simulink model "vehicle_model"  (R2021b)
settings: Solver=ode23tb  StartTime=0  StopTime=2474  FixedStep=1e-5  RelTol=2e-1
InitFcn:
  | param_v1_script;
  | Ts=0.01;
  | scenario_generator;
  | Regen_on=1;
  | v_nom=10;
values from neighbouring files (symbols this model uses):
  b = 1.504    [dynamics_wheel.m]    (also in param_v1_script.m = Simulink.Parameter)
  BattChargeMax = 4.8    [param_v1_script.m]
  Battery = struct    [param_v1_script.m]
  BattSocInit = 0.75    [param_v1_script.m]
  BattTempInit = 25    [param_v1_script.m]
  BrkPrsMax = 5.0E+6    (= 5000000)    [param_v1_script.m]
  car = vehicle(scenario,'ClassID',1,'Position',[x_ego y_ego 0], 'Yaw' ,0,     'Length',3,'Width',2,'Height',1.6)    [scenario_generator.m]
  disk_abore = 0.05    [param_v1_script.m]
  Eb_init = 54.28*1000*3600    (= 195408000)    [param_v1_script.m]
  efficiency_table = [86.7 86.7 86.7 86.7 86.7 86.7 86.7 86.7 86.7 86.7 86.7 86.7 86.7 86.7     86.7 ... (first row only)    [param_v1_script.m]
  eta_i = 1    [param_v1_script.m]
  Jmotor = Simulink.Parameter    [param_v1_script.m]
  k = Simulink.Parameter    [param_v1_script.m]
  L = 30000    [scenario_generator.m]
  losses_table = [0 0 0 0 0 0 0 0 0 0 0 0 0 0 0 ... (first row only)    [param_v1_script.m]
  m = VEH.Mass    [param_v1_script.m]
  MaxChrgCurrLim = Simulink.Parameter    [param_v1_script.m]
  MaxDchrgCurrLim = Simulink.Parameter    [param_v1_script.m]
  MinCellVoltDchrgCurrentLim_BP = [2.5; 2.75; 3]    [param_v1_script.m]
  MinCellVoltDchrgCurrentLim_Table = [0 0.5 1]    [param_v1_script.m]
  MotSpd = [0 1600 3200 4477.56 4800 6400 8000 9600 11200 12800 14400 16000            ]    [param_v1_script.m]
  MotTrq = [450 450 450 450 419.771162404874 314.828371803655 251.862697442924            209.885581202437 179.901926744946 157.414185901828 139.923720801625            125.931348721462]    [param_v1_script.m]
  mu_kinetic = 0.2    [param_v1_script.m]
  Nd = 7.94    [param_v1_script.m]
  Ndiff = Simulink.Parameter    [param_v1_script.m]
  Np_Module = 31    [param_v1_script.m]
  Ns_Module = 24    [param_v1_script.m]
  num_pads = 2    [param_v1_script.m]
  NumModules = 4    [param_v1_script.m]
  RegenBrkCutOff = [0 1]    [param_v1_script.m]
  RegenBrkSpd_bpt = [5 9]    [param_v1_script.m]
  Rm = 0.177    [param_v1_script.m]
  rw = 0.3345    [param_v1_script.m]
  scenario = drivingScenario('SampleTime',0.1','StopTime',60)    [scenario_generator.m]
  SOCInit = 0.75    [param_v1_script.m]
  SOE_init = SOCInit    (= 0.75)    [param_v1_script.m]
  T_eff_bp = [0 32.142857142857146 64.285714285714292 96.428571428571431              128.57142857142858 160.71428571428572 192.85714285714286 225              257.14285714285717 289.28571428571428 321.42857142857144 353.57142857142856              385.71428571428572 417.85714285714283 450]    [param_v1_script.m]
  threshld = 50    [scenario_generator.m]
  VEH = struct    [dynamics_wheel.m]
  w_eff_bp = [0 1600 3200 4477.56 4800 6400 8000 9600 11200 12800 14400 16000              ]    [param_v1_script.m]
undefined symbols (not defined in the file or in its folder): curvature, direction, DiscIntNeverNeededParam, gradbp, InertFrm, psi_o, thetaRefs, xRef2s, yRef2s
libraries: simulink x11, autolibutils x4, autolibshared x4, autolibsharedcoupling x4, sharedtransform x3, vehdynlibdriver x3, simulink_extras x3, sharedTrackingLibrary x2, vehdynlibtirecommon x2, vehdynlibtire x2, vehdynlibdrivercommon x2, vehdynlibscenariocommon x1
(part 1 of 6)
settings Model: Creator=simran  LastModifiedBy=simran
settings SolverCC: ZeroCrossAlgorithm=Adaptive
settings DebuggingCC: MaskedZcDiagnostic=none  IgnoredZcDiagnostic=none

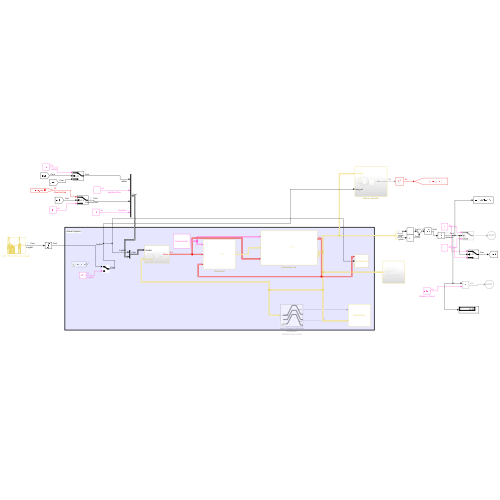
[thumbnail: Simulink's stored preview of the top-level diagram]
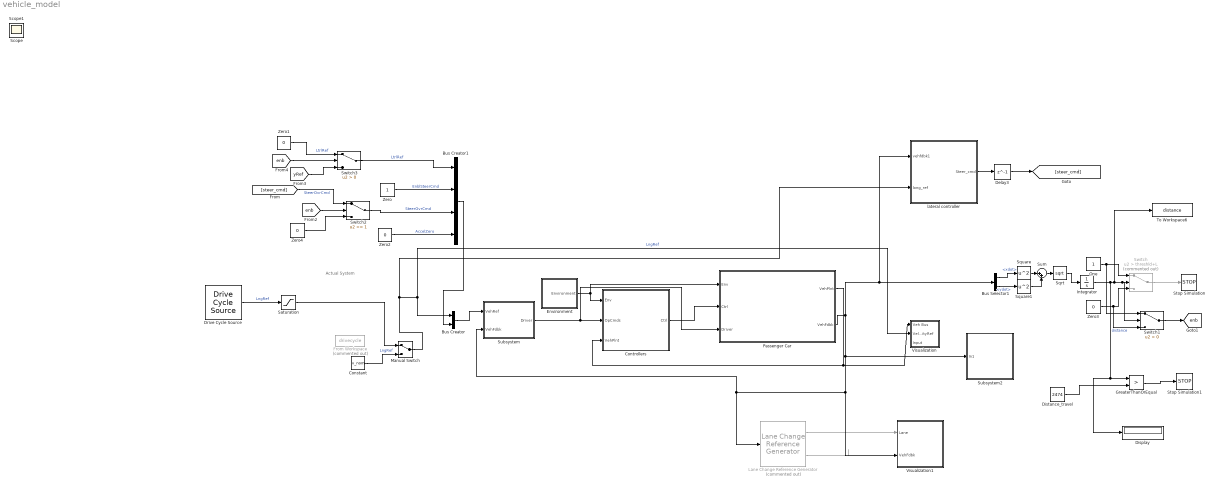
== system vehicle_model ==
  note: Actual System
  Bus Creator : BusCreator  Inputs=2
  Bus Creator1 : BusCreator  Inputs=4
  Bus Selector1 : BusSelector  OutputSignals=Body.BdyFrm.Cg.Vel.xdot,Body.BdyFrm.Cg.Vel.ydot
  Constant : Constant  Value=v_nom
  Controllers : Subsystem
      mask Display: image('SystemControllers.png','center')
  Delay3 : Delay  DelayLength=1
  Display : Display
  Distance_travel : Constant  Value=2474
  Drive Cycle Source : autolibshared/Drive Cycle Source  cycleVar=FTP75  fileVar=L:\Bauto\matlab\test\toolbox\shared\autoblks\scenario\adac.txt  tfinal="2474  seconds"  cycleRepeat=off  outAccPort=off  outGearPort=off  gearList=No gear data  t_wot1=1  xdot_woto=0  xdot_wot1=26.8*1.1  t_wot2=30  xdot_wot2=0  t_wotend=40  srcUnit=m/s  outUnit=m/s  srcAccUnit=m/s/s  outAccUnit=m/s^2  dt=0  aMode=1  faultOption=off  velBnd=2  velBndUnit=mph  inUnit=m/s  timeBnd=1  failOption=off  stopSim=off  maxFaultCnt=10  maxFaultTime=2  maxTotFaultTime=15  traceOption=off  dtTrace=1  traceWindow=10  lastDCname=FTP75  lastOutUnit=mph  lastDT=0  lastTB=1  lastSB=2  forceCalcBound=off
      settings: SourceProductBaseCode=PW,DR,MT,UV,VE
  Environment : Subsystem
      mask Display: disp(getString(message('autoblks:autoblkVehMask:environ')))
  From Workspace : FromWorkspace  Commented=on  VariableName=drivecycle  SampleTime=-1
  GreaterThanOrEqual : RelationalOperator  Operator=>  OutDataTypeStr=boolean  RndMeth=Simplest
  Integrator : Integrator
  Lane Change Reference Generator : vehdynlibscenariocommon/Lane Change Reference Generator  Commented=on  ssMode=Initialize from model  ssVar=dlcSS35mph  t_start=1  XGate=200  xdot_r=35  xdotUnit=mph  xStart=2  vehW=2  latoff=800  lattoff=VEH.InitialLatPosition  centerSwitch=on  xSimStop=off  ssDefault=on  latRefbp=DLCXref  latRef=DLCYref  X_o=175  Y_o=VEH.InitialLatPosition  psi_o=VEH.InitialYawAngle  ssTol=.15  ssMaxTime=30  ssWSName=dlcSS35mph  aMode=2
      link override ISO 3888-2/Lateral Reference: LabelModeActiveChoice=1
      settings: AttributesFormatString=%<ssMode>  SourceProductBaseCode=VE
  Manual Switch : ManualSwitch
  One : Constant  OutDataTypeStr=Inherit: Inherit via back propagation
  Passenger Car : Subsystem
      mask Display: image('PassengerVehicle.png','center')
  Saturation : Saturate  UpperLimit=inf  LowerLimit=5
  Sqrt : Sqrt  SaturateOnIntegerOverflow=on
  Square : Math  Operator=square  SaturateOnIntegerOverflow=on
  Square1 : Math  Operator=square  SaturateOnIntegerOverflow=on
  Stop Simulation : Stop
  Stop Simulation1 : Stop
  Subsystem : Subsystem
  Subsystem2 : Subsystem
  Sum : Sum  Inputs=|++
  Switch : Switch  Commented=on  Criteria=u2 > Threshold  Threshold=threshld+L
  Switch1 : Switch  Criteria=u2 > Threshold
  Switch2 : Switch  Threshold=1
  Switch3 : Switch  Criteria=u2 > Threshold
  To Workspace6 : ToWorkspace  VariableName=distance  SaveFormat=Timeseries  SampleTime=-1
  Visualization : Subsystem
      mask Display: disp(getString(message('autoblks:autoblkVehMask:visual')))
  Visualization1 : Subsystem
      mask Display: disp('Visualization')
  Zero : Constant  OutDataTypeStr=Inherit: Inherit via back propagation
  Zero{1..4} (4 alike) : Constant  Value=0  OutDataTypeStr=Inherit: Inherit via back propagation
  lateral controller : Subsystem
  Scope : Scope
  Scope1 : Scope
  tag scope: enb=global
  wires:
  Lane Change Reference Generator/2 -> ?
  [yRef] -> Switch3/3
  Delay3/1 -> [steer_cmd]
  One/1 -> Switch1/1, Switch/1
  [enb] -> Switch3/2
  Switch1/1 -> [enb]
  lateral controller/1(Steer_cmd) -> Delay3/1
  Integrator/1 -> To Workspace6/1, Switch1/2, Switch/2, Display/1, GreaterThanOrEqual/1  "distance"
  Switch2/1 -> Bus Creator1/3  "SteerOvrCmd"
  Bus Creator1/1 -> Bus Creator/2
  Zero/1 -> Bus Creator1/2  "EnblSteerCmd"
  Bus Creator/1 -> Subsystem/1(VehRef)
  Zero2/1 -> Bus Creator1/4  "AccelZero"
  Switch3/1 -> Bus Creator1/1  "LtrlRef"
  Zero3/1 -> Switch1/3, Switch/3
  Lane Change Reference Generator/1 -> Visualization1/1(Lane)
  Switch/1 -> Stop Simulation/1
  Zero4/1 -> Switch2/3
  Environment/1(Environment) -> Controllers/1(Env), Passenger Car/1(Env)
  Bus Selector1/1 -> Square/1  "<xdot>"
  Passenger Car/2(VehFdbk) -> lateral controller/1(vehfdbk1), Bus Selector1/1, Subsystem/2(VehFdbk), Lane Change Reference Generator/1, Visualization1/2(VehFdbk), Subsystem2/1(In1)
  Manual Switch/1 -> lateral controller/2(long_ref), Visualization/2(VelocityRef), Bus Creator/1  "LngRef"
  Controllers/1(Ctrl) -> Passenger Car/2(Ctrl)
  Zero1/1 -> Switch3/1  "LtrlRef"
  [enb] -> Switch2/2
  Passenger Car/1(VehPlnt) -> Controllers/3(VehPlnt), Visualization/1(Veh Bus)
  Bus Selector1/2 -> Square1/1  "<ydot>"
  Square/1 -> Sum/1
  Square1/1 -> Sum/2
  Sum/1 -> Sqrt/1
  Sqrt/1 -> Integrator/1
  Distance_travel/1 -> GreaterThanOrEqual/2
  GreaterThanOrEqual/1 -> Stop Simulation1/1
  Subsystem/1(Driver) -> Passenger Car/3(Driver), Controllers/2(OpCmds)
  Constant/1 -> Manual Switch/2  "LngRef"
  Drive Cycle Source/1 -> Saturation/1  "LngRef"
  Saturation/1 -> Manual Switch/1
  [steer_cmd] -> Switch2/1  "SteerOvrCmd"

== system vehicle_model/Controllers ==
  Env : Inport
  OpCmds : Inport  Port=2
  VehPlnt : Inport  Port=3
  Powertrain Control Input : Subsystem
  Powertrain Control Module (PCM) : Subsystem
  Powertrain Control Output : Subsystem
  Terminator : Terminator
  Ctrl : Outport  VectorParamsAs1DForOutWhenUnconnected=off
  wires:
  [PtCtrl] -> Ctrl/1
  Env/1 -> Terminator/1
  [OpCmds] -> Powertrain Control Input/1(OpCmds)
  Powertrain Control Output/1(PtCtrl) -> [PtCtrl]
  [VehPlnt] -> Powertrain Control Input/2(VehPlnt)
  VehPlnt/1 -> [VehPlnt]
  OpCmds/1 -> [OpCmds]
  Powertrain Control Input/1(AccelPdl) -> Powertrain Control Module (PCM)/1(AccCmd)
  Powertrain Control Input/2(DecelPdl) -> Powertrain Control Module (PCM)/2(DecCmd)
  Powertrain Control Input/3(VehSpdFdbk) -> Powertrain Control Module (PCM)/3(VehSpdFdbk)
  Powertrain Control Input/4(MotSpd) -> Powertrain Control Module (PCM)/4(MotSpd)
  Powertrain Control Module (PCM)/1(MotTrqCmd) -> Powertrain Control Output/1(MotTrqCmd)
  Powertrain Control Module (PCM)/2(BrakeCmd) -> Powertrain Control Output/2(BrkCmd)
  Powertrain Control Input/5(BMS_Sensors) -> Powertrain Control Module (PCM)/5(BMS_Sensors)
  Powertrain Control Module (PCM)/3(BMS_Info) -> Powertrain Control Output/3(BMS_Info)
  Powertrain Control Module (PCM)/4(BMS_Cmd) -> Powertrain Control Output/4(BMS_Cmd)

== system vehicle_model/Environment ==
  Bus Creator : BusCreator  Inputs=4
  Bus Creator1 : BusCreator  Inputs=4
  Bus Creator2 : BusCreator  Inputs=4
  Bus Creator3 : BusCreator  Inputs=3
  Bus Creator4 : BusCreator  Inputs=3
  Bus Creator5 : BusCreator  Inputs=2
  Constant : Constant  Value=zeros(4,1)
  Constant1 : Constant  Value=ones(4,1)
  Constant2 : Constant  Value=0
  Constant3 : Constant  Value=0
  Constant6 : Constant  Value=300
  Constant7 : Constant  Value=101325
  Demux : Demux
  Demux1 : Demux
  Ground{,1..3} (4 alike) : Ground
  Environment : Outport  VectorParamsAs1DForOutWhenUnconnected=off
  wires:
  Ground2/1 -> Bus Creator5/1  "lam_mu_x"
  Ground3/1 -> Bus Creator5/2  "lam_mu_y"
  Bus Creator2/1 -> Bus Creator4/2  "Ground_mu"
  Bus Creator4/1 -> Bus Creator/3  "Ground"
  Bus Creator3/1 -> Bus Creator/4  "Wind"
  Constant3/1 -> Bus Creator3/1  "wind_x"
  Ground/1 -> Bus Creator3/2  "wind_y"
  Ground1/1 -> Bus Creator3/3  "wind_z"
  Constant6/1 -> Bus Creator/1  "Temp"
  Constant2/1 -> Bus Creator4/1  "Grade"
  Bus Creator/1 -> Environment/1  "Environment"
  Constant7/1 -> Bus Creator/2  "Baro"
  Constant/1 -> Demux/1
  Demux/1 -> Bus Creator1/1  "G_FL_z"
  Demux/2 -> Bus Creator1/2  "G_FR_z"
  Demux/3 -> Bus Creator1/3  "G_RL_z"
  Demux/4 -> Bus Creator1/4  "G_RR_z"
  Bus Creator1/1 -> Bus Creator4/3  "z"
  Constant1/1 -> Demux1/1
  Demux1/1 -> Bus Creator2/1  "mu_FL"
  Demux1/2 -> Bus Creator2/2  "mu_FR"
  Demux1/3 -> Bus Creator2/3  "mu_RL"
  Demux1/4 -> Bus Creator2/4  "mu_RR"

== system vehicle_model/Passenger Car ==
  Env : Inport
  Ctrl : Inport  Port=2
  Driver : Inport  Port=3
  Bus Creator : BusCreator  Inputs=2
  Drivetrain Output : Subsystem
  Drivetrain Plant Input : Subsystem
  Electric Plant Input : Subsystem
  Electric Plant Output : Subsystem
  Subsystem : Subsystem
  Subsystem1 : Subsystem
  Zero-Order Hold : ZeroOrderHold  SampleTime=0.01
  VehPlnt : Outport  VectorParamsAs1DForOutWhenUnconnected=off
  Bus Element Out1 : Outport  Port=2  PortName=VehFdbk  Element=Body
  Bus Element Out2 : Outport  Port=2  PortName=VehFdbk  Element=Wheels
  wires:
  Ctrl/1 -> [Ctrl]
  Env/1 -> [Env], Electric Plant Input/3(Env)  "Env"
  [Ctrl] -> Drivetrain Plant Input/1(Ctrl)
  [VehFdbk] -> Bus Creator/2  "Veh"
  [ElecFdbk] -> Bus Creator/1  "Elec"
  [Ctrl] -> Electric Plant Input/1(Ctrl)  "Ctrl"
  [ElecFdbk] -> Drivetrain Plant Input/2(ElecFdbk)
  [VehFdbk] -> Electric Plant Input/2(Veh)  "Vehfdbk"
  Drivetrain Plant Input/2(BrkCmd) -> Subsystem1/2(BrakeReq)
  Drivetrain Plant Input/1(MotTrq) -> Subsystem1/1(MotTrq)
  Subsystem1/2(MotSpd) -> Drivetrain Output/2(MotSpd)
  Subsystem1/1(vel) -> Drivetrain Output/1(Vel)
  [Env] -> Drivetrain Plant Input/3(Env)
  Drivetrain Plant Input/3(Grade) -> Subsystem1/3(Grade)
  Drivetrain Plant Input/4(WindVel) -> Subsystem1/4(Wind Vel)
  Electric Plant Input/1(MotTrqCmd) -> Subsystem/1(MotTrqCmd)
  Electric Plant Input/2(MotSpd) -> Subsystem/2(MotSpd)
  Electric Plant Input/3(AmbTmp) -> Subsystem/3(AmbTmp)
  Subsystem/2(BattPwr) -> Electric Plant Output/2(BattPwr)
  Subsystem/3(BattCrnt) -> Electric Plant Output/3(BattCrnt)
  Subsystem/4(MotTrq) -> Electric Plant Output/4(MotTrq)
  Subsystem/5(BMS_Sensors) -> Electric Plant Output/5(BMS_Sensors)
  Electric Plant Input/4(BMS_Info) -> Subsystem/4(BMS_Info)
  Subsystem/1(BattSoc) -> Electric Plant Output/1(BattSoc)
  Drivetrain Plant Input/5(mu) -> Subsystem1/5(mu)
  Drivetrain Plant Input/6(Gnd) -> Subsystem1/6(Ground)
  Electric Plant Output/1(ElecFdbk) -> [ElecFdbk]  "Elecfdbk"
  Subsystem1/3(Veh) -> Bus Element Out1/1
  Driver/1 -> Drivetrain Plant Input/4(Driver)  "Drive_input"
  Drivetrain Plant Input/7(Steer) -> Subsystem1/7(Steering)
  Subsystem1/4(Wheels) -> Bus Element Out2/1
  Bus Creator/1 -> Zero-Order Hold/1
  Drivetrain Output/1(VehFdbk) -> [VehFdbk]
  Zero-Order Hold/1 -> VehPlnt/1

== system vehicle_model/Subsystem ==
  VehRef : Inport
  VehFdbk : Inport  Port=2
  Bus Creator1 : BusCreator  Inputs=5
  Bus Selector : BusSelector  OutputSignals=Body.BdyFrm.Cg.Vel.xdot,Body.InertFrm.Cg.Disp.Y,Body.BdyFrm.Cg.Vel.ydot,Body.InertFrm.Cg.Ang.psi,Body.BdyFrm.Cg.AngVel.r,Body.InertFrm.Cg.Disp.X
  Bus Selector1 : BusSelector  OutputSignals=LngRef,signal2.LtrlRef,signal2.EnblSteerCmd,signal2.SteerOvrCmd,signal2.AccelZero
  Cast To Boolean : DataTypeConversion  OutDataTypeStr=boolean
  Constant : Constant  Value=0
  Dead Zone : DeadZone  LowerValue=-.5  UpperValue=.5  ZeroCross=off  SaturateOnIntegerOverflow=on
  From Workspace : FromWorkspace  Commented=on  VariableName=acel  SampleTime=-1
  From Workspace1 : FromWorkspace  Commented=on  VariableName=dcel  SampleTime=-1
  Gain : Gain
  Ground : Ground
  Ground1 : Ground
  Ground2 : Ground
  Longitudinal Driver : autolibshared/Longitudinal Driver  extAccelOvr=off  extDecelOvr=off  extAccelHld=off  extDecelHld=off  extAccelZero=off  extDecelZero=off  cntrlType=PI  shftType=None  velUnits=m/s  gearOut=off  Kp=10  Ki=5  Kff=.1  Kg=0  VehVelVec=[0 100]  KffVec=[.1 .1]  KpVec=[10 10]  KiVec=[5 5]  KgVec=[0 0]  m=1500  Kpt=3000  tau=.1  L=2  aR=200  bR=2.5  cR=.5  g=9.81  vnom=10  Kaw=1  tauerr=.01  tauPt=2  GearInit=0  tShift=.1  pdlVec=[0.1 0.4 0.5 0.9]  upShftTbl=[-1 12.9375 26.4375 39.9375 51.18749999999999 62.4375 72.84375 83.25;-1 16.3125 29.8125 43.3125 54.5624 65.8125 76.78125 87.75;-1 19.6875 33.1875 46.68749999999999 57.9375 69.1875 80.71875 92.25;-1 33 52.5 77.25 100.5 138.75 161.875 185]  dwnShftTbl=[1 9.5625 23.0625 36.5625 47.8125 59.0625 68.90625 78.75;1 12.9375 26.4375 39.9375 51.18749999999999 62.4375 72.84375 83.25;1 16.3125 29.8125 43.3125 54.562499 65.8125 76.78125 87.75;1 19.6875 33.1875 46.68749999999999 57.9375 69.1875 80.71875 92.25]  tClutch=.5  tRev=.5  tPark=120  aMode=2  UpGearVec="[0  1  2  3  4  5  6  7]"  DownGearVec="[1  2  3  4  5  6  7  8]"
      settings: SourceProductBaseCode=PW,DR,MT,UV,VE
  Mux : Mux  Inputs=3
  Subsystem : Subsystem  Commented=on
  Terminator1 : Terminator
  Terminator2 : Terminator
  Zero : Constant  Value=0  OutDataTypeStr=Inherit: Inherit via back propagation
  Zero-Order Hold : ZeroOrderHold  SampleTime=Ts
  Zero1 : Constant  Value=0  OutDataTypeStr=Inherit: Inherit via back propagation
  Driver : Outport  VectorParamsAs1DForOutWhenUnconnected=off
  wires:
  Dead Zone/1 -> Longitudinal Driver/2, Subsystem/6(VelFdbk)
  Bus Selector1/1 -> Subsystem/1(VelRef), Longitudinal Driver/1  "<LngRef>"
  Bus Selector1/4 -> Gain/1, Subsystem/3(SteerOvrCmd)  "<SteerOvrCmd>"
  Bus Selector1/3 -> Subsystem/4(EnblSteerOvr)  "<EnblSteerCmd>"
  VehRef/1 -> Bus Selector1/1  "xdotref"
  VehFdbk/1 -> Bus Selector/1
  Zero1/1 -> Mux/3
  Longitudinal Driver/2 -> Bus Creator1/2  "AccelCmd"
  Bus Selector/3 -> Subsystem/8(LatVelFdbk)  "<ydot>"
  Bus Selector/4 -> Subsystem/9(YawFdbk)  "<psi>"
  Zero/1 -> Subsystem/7(LatFdbk)
  Bus Creator1/1 -> Zero-Order Hold/1
  Bus Selector/5 -> Subsystem/10(YawVelFdbk)  "<r>"
  Ground/1 -> Subsystem/5(Grade)
  Longitudinal Driver/3 -> Bus Creator1/3  "DecelCmd"
  Bus Selector/1 -> Dead Zone/1  "<xdot>"
  Bus Selector1/2 -> Subsystem/2(LatRef), Mux/2  "<LtrlRef>"
  Ground2/1 -> Bus Creator1/4  "GearCmd"
  Bus Selector/6 -> Mux/1  "<X>"
  Mux/1 -> Bus Creator1/5  "Ref"
  Subsystem/1(Info) -> Terminator1/1
  Constant/1 -> Cast To Boolean/1
  Ground1/1 -> Longitudinal Driver/3
  Longitudinal Driver/1 -> Terminator2/1
  Gain/1 -> Bus Creator1/1  "SteerCmd"
  Zero-Order Hold/1 -> Driver/1

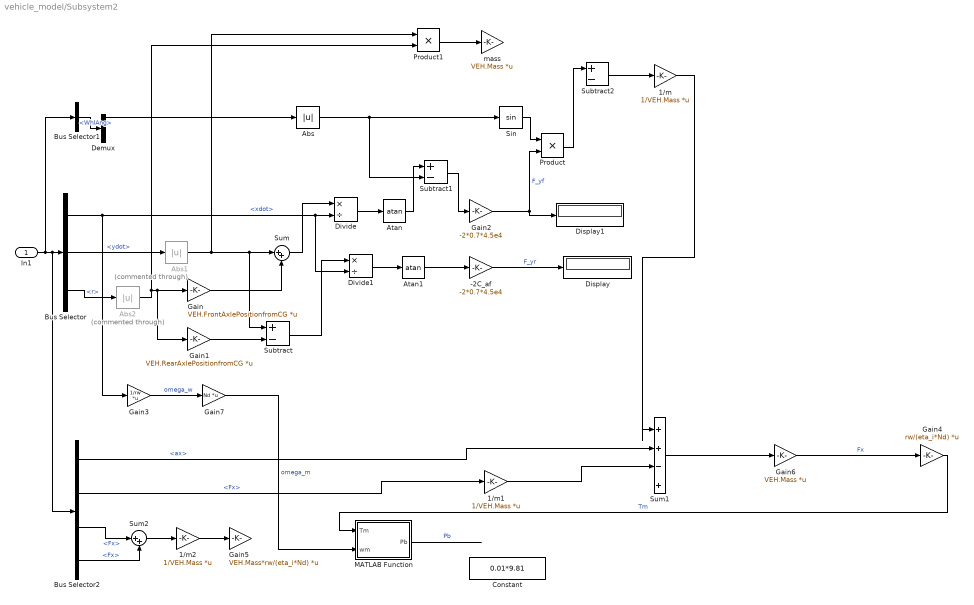
== system vehicle_model/Subsystem2 ==
  In1 : Inport
  -2C_af : Gain  Gain=-2*0.7*4.5e4
  1/m : Gain  Gain=1/VEH.Mass  Multiplication=Matrix(K*u)
  1/m1 : Gain  Gain=1/VEH.Mass  Multiplication=Matrix(K*u)
  1/m2 : Gain  Gain=1/VEH.Mass  Multiplication=Matrix(K*u)
  Abs : Abs
  Abs1 : Abs  Commented=through
  Abs2 : Abs  Commented=through
  Atan : Trigonometry  Operator=atan
  Atan1 : Trigonometry  Operator=atan
  Bus Selector : BusSelector  OutputSignals=Body.BdyFrm.Cg.Vel.xdot,Body.BdyFrm.Cg.Vel.ydot,Body.BdyFrm.Cg.AngVel.r
  Bus Selector1 : BusSelector  OutputSignals=Wheels.signal1.Steering.WhlAng
  Bus Selector2 : BusSelector  OutputSignals=Body.BdyFrm.Cg.Acc.ax,Body.BdyFrm.Forces.Drag.Fx,Body.BdyFrm.Forces.RearAxl.Lft.Fx,Body.BdyFrm.Forces.RearAxl.Rght.Fx
  Constant : Constant  Value=0.01*9.81
  Demux : Demux
  Display : Display
  Display1 : Display
  Divide : Product  Inputs=*/
  Divide1 : Product  Inputs=*/
  Gain : Gain  Gain=VEH.FrontAxlePositionfromCG  Multiplication=Matrix(K*u)
  Gain1 : Gain  Gain=VEH.RearAxlePositionfromCG  Multiplication=Matrix(K*u)
  Gain2 : Gain  Gain=-2*0.7*4.5e4
  Gain3 : Gain  Gain=1/rw  Multiplication=Matrix(K*u)
  Gain4 : Gain  Gain=rw/(eta_i*Nd)  Multiplication=Matrix(K*u)
  Gain5 : Gain  Gain=VEH.Mass*rw/(eta_i*Nd)  Multiplication=Matrix(K*u)
  Gain6 : Gain  Gain=VEH.Mass  Multiplication=Matrix(K*u)
  Gain7 : Gain  Gain=Nd  Multiplication=Matrix(K*u)
  MATLAB Function : MATLAB Function  TreatAsAtomicUnit=on
  Product : Product
  Product1 : Product
  Sin : Trigonometry
  Subtract : Sum  Inputs=+-
  Subtract1 : Sum  Inputs=+-
  Subtract2 : Sum  Inputs=+-
  Sum : Sum  Inputs=|++
  Sum1 : Sum  Inputs=|++-+
  Sum2 : Sum  Inputs=|++
  mass : Gain  Gain=VEH.Mass  Multiplication=Matrix(K*u)
  wires:
  In1/1 -> Bus Selector1/1, Bus Selector2/1, Bus Selector/1
  Bus Selector/2 -> Abs1/1  "<ydot>"
  Bus Selector/3 -> Abs2/1  "<r>"
  Gain/1 -> Sum/2
  Gain1/1 -> Subtract/2
  Sum/1 -> Divide/1
  Bus Selector/1 -> Gain3/1, Divide/2, Divide1/2  "<xdot>"
  Subtract/1 -> Divide1/1
  Divide/1 -> Atan/1
  Divide1/1 -> Atan1/1
  Atan1/1 -> -2C_af/1
  Atan/1 -> Subtract1/1
  Gain2/1 -> Product/2, Display1/1  "F_yf"
  -2C_af/1 -> Display/1  "F_yr"
  Bus Selector1/1 -> Demux/1  "<WhlAng>"
  Demux/1 -> Abs/1
  Subtract1/1 -> Gain2/1
  Gain7/1 -> MATLAB Function/2(wm)  "omega_m"
  Sin/1 -> Product/1
  Product1/1 -> mass/1
  Product/1 -> Subtract2/1
  Subtract2/1 -> 1/m/1
  1/m1/1 -> Sum1/3
  Bus Selector2/1 -> Sum1/2  "<ax>"
  1/m/1 -> Sum1/1
  Sum1/1 -> Gain6/1
  Bus Selector2/3 -> Sum2/1  "<Fx>"
  Bus Selector2/4 -> Sum2/2  "<Fx>"
  Sum2/1 -> 1/m2/1
  1/m2/1 -> Gain5/1
  Gain4/1 -> MATLAB Function/1(Tm)  "Tm"
  MATLAB Function/1(Pb) -> ?  "Pb"
  Abs/1 -> Sin/1, Subtract1/2
  Abs1/1 -> Product1/1, Subtract/1, Sum/1
  Abs2/1 -> Gain1/1, Gain/1, Product1/2
  Gain3/1 -> Gain7/1  "omega_w"
  Bus Selector2/2 -> 1/m1/1  "<Fx>"
  Gain6/1 -> Gain4/1  "Fx"

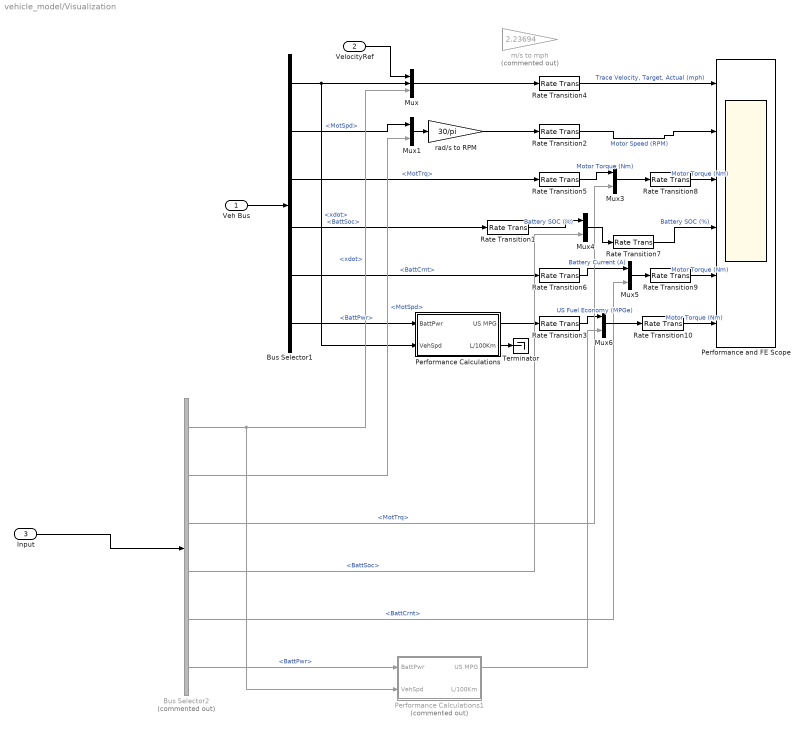
== system vehicle_model/Visualization ==
  Veh Bus : Inport
  VelocityRef : Inport  Port=2
  Input : Inport  Port=3
  Bus Selector1 : BusSelector  OutputSignals=Veh.xdot,Veh.MotSpd,Elec.MotTrq,Elec.BattSoc,Elec.BattCrnt,Elec.BattPwr
  Bus Selector2 : BusSelector  Commented=on  OutputSignals=Veh.xdot,Veh.MotSpd,Elec.MotTrq,Elec.BattSoc,Elec.BattCrnt,Elec.BattPwr
  Mux : Mux  Inputs=3
  Mux{1,3..6} (5 alike) : Mux  Inputs=2
  Performance Calculations : Subsystem
  Performance Calculations1 : Subsystem  Commented=on
  Performance and FE Scope : Scope  NumInputPorts=6
  Rate Transition{1..10} (10 alike) : RateTransition  Deterministic=off
  Terminator : Terminator
  m/s to mph : Gain  Commented=on  Gain=2.23694
  rad/s to RPM : Gain  Gain=30/pi
  wires:
  Veh Bus/1 -> Bus Selector1/1
  Bus Selector1/1 -> Performance Calculations/2(VehSpd), Mux/2  "<xdot>"
  Performance Calculations/1(US MPG) -> Rate Transition3/1
  Performance Calculations/2(L/100Km) -> Terminator/1
  Mux/1 -> Rate Transition4/1
  Bus Selector1/4 -> Rate Transition1/1  "<BattSoc>"
  VelocityRef/1 -> Mux/1
  Rate Transition1/1 -> Mux4/1  "Battery SOC (%)"
  Rate Transition2/1 -> Performance and FE Scope/2  "Motor Speed (RPM)"
  Rate Transition4/1 -> Performance and FE Scope/1  "Trace Velocity, Target, Actual (mph)"
  Bus Selector1/2 -> Mux1/1  "<MotSpd>"
  Bus Selector1/6 -> Performance Calculations/1(BattPwr)  "<BattPwr>"
  rad/s to RPM/1 -> Rate Transition2/1
  Bus Selector1/3 -> Rate Transition5/1  "<MotTrq>"
  Rate Transition5/1 -> Mux3/1  "Motor Torque (Nm)"
  Rate Transition6/1 -> Mux5/1  "Battery Current (A)"
  Bus Selector1/5 -> Rate Transition6/1  "<BattCrnt>"
  Rate Transition3/1 -> Mux6/1  "US Fuel Economy (MPGe)"
  Input/1 -> Bus Selector2/1
  Bus Selector2/1 -> Performance Calculations1/2(VehSpd), Mux/3  "<xdot>"
  Bus Selector2/2 -> Mux1/2  "<MotSpd>"
  Mux3/1 -> Rate Transition8/1
  Bus Selector2/3 -> Mux3/2  "<MotTrq>"
  Mux4/1 -> Rate Transition7/1
  Bus Selector2/4 -> Mux4/2  "<BattSoc>"
  Mux5/1 -> Rate Transition9/1
  Bus Selector2/5 -> Mux5/2  "<BattCrnt>"
  Mux6/1 -> Rate Transition10/1
  Mux1/1 -> rad/s to RPM/1
  Bus Selector2/6 -> Performance Calculations1/1(BattPwr)  "<BattPwr>"
  Performance Calculations1/1(US MPG) -> Mux6/2
  Rate Transition7/1 -> Performance and FE Scope/4  "Battery SOC (%)"
  Rate Transition8/1 -> Performance and FE Scope/3  "Motor Torque (Nm)"
  Rate Transition9/1 -> Performance and FE Scope/5  "Motor Torque (Nm)"
  Rate Transition10/1 -> Performance and FE Scope/6  "Motor Torque (Nm)"

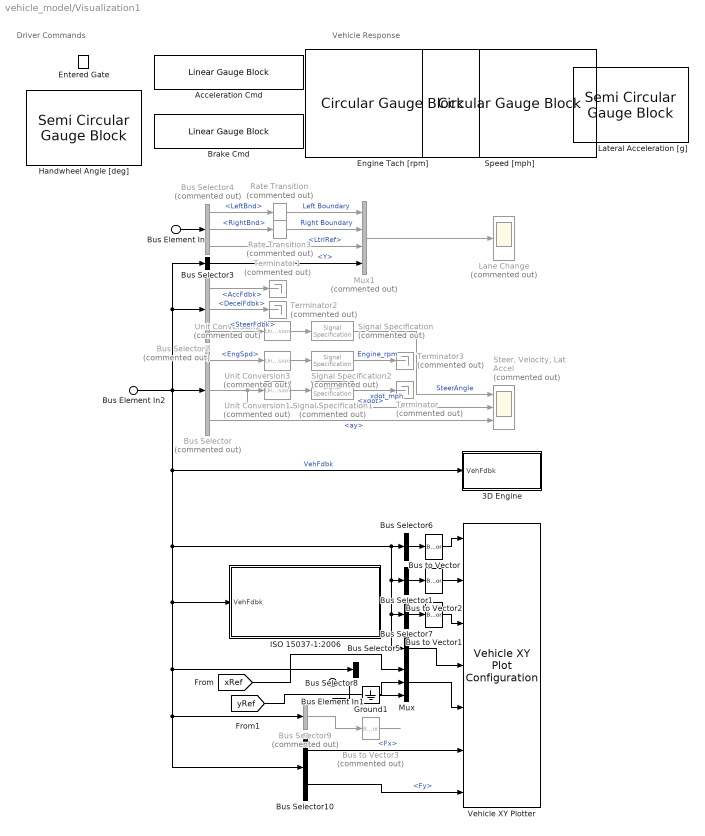
== system vehicle_model/Visualization1 ==
  note: Vehicle Response
  note: Driver Commands
  Bus Element In : Inport  PortName=Lane
  Bus Element In1 : Inport  PortName=Lane  Element=LtrlRef
  Bus Element In2 : Inport  Port=2  PortName=VehFdbk
  3D Engine : Subsystem  Variant=on  mask(3D Engine){engine3D=Disabled, use3DOp=off, SceneDesc=Double lane change, dt3D=.03, defaultPos=Recommended for scene, X_o=0, Y_o=3.125, Z_o=0, phi_o=0, theta_o=0, psi_o=0}
      mask prompts: engine3D "3D Engine"; use3DOp "Use default operating point"; SceneDesc "Scene:"; dt3D "Engine frame rate, dt3D [s]:"; X_o "Initial longitudinal position, X_o [m]:"; Y_o "Initial lateral position, Y_o [m]:"; Z_o "Initial vertical position, Z_o [m]:"; phi_o "Initial roll angle, phi_o [rad]:"; theta_o "Initial pitch angle, theta_o [rad]:"; psi_o "Initial yaw angle, psi_o [rad]:"
      mask help: This subsystem contains the interface blocks which permit the display of the vehicle in the 3D virtual environment. Enable it to view the simulation progress, disable it to inhibit the display.
      mask init:
      | switch get_param(gcb,'engine3D')
      |     case 'Disabled'
      |         try
      |             set_param([bdroot '/Environment/Ground Feedback'],'OverrideUsingVariant','0');
      |         catch
      |             disp('Warning: No ground feedback sensor not set')
      |         end
      |         try
      |             if strcmp(get_param(gcb,'use3DOp'),'on') && strcmp(get_param('DLCReferenceApplication/Lane Change Reference Generator','ssMode'),'Resume from a workspace variable')
      |                 set_param('DLCReferenceApplication/Lane Change Reference Generator','ssVar','dlcSS35mph');
      |             end
      |         catch
      |              disp('Warning: Lane Change Reference Generator not found. Steady state operating point not set')
      |         end
      |     case 'Enabled'
      |         try
      |             set_param([bdroot '/Environment/Ground Feedback'],'OverrideUsingVariant','1');            
      |         catch
      |             disp('Warning: No ground feedback sensor not set')
      |         end
      |         try
      |             if strcmp(get_param(gcb,'use3DOp'),'on') && strcmp(get_param('DLCReferenceApplication/Lane Change Reference Generator','ssMode'),'Resume from a workspace variable')
      |                 set_param('DLCReferenceApplication/Lane Change Reference Generator','ssVar','dlcSS35mph3D');
      |             end
      |         catch
      |              disp('Warning: Lane Change Reference Generator not found. Steady state operating point not set')
      |         end
      |     otherwise
      | end
      settings: AttributesFormatString=|
      | %<SceneDesc>
      | %<engine3D>
      mask Help: eval('vdynblkshelp(''vdynblks3dengine'')');
      mask TypeOptions engine3D: Enabled | Disabled
      mask TypeOptions SceneDesc: 3D Engine/Simulation 3D Scene Configuration/SceneDesc
      mask Callback SceneDesc:
      | defaultStatus = get_param(gcb,'defaultPos');
      | if strcmp(defaultStatus,'Recommended for scene')
      | sceneType = get_param(gcb,'SceneDesc');
      | switch sceneType
      |     case 'Straight road'
      |         set_param(gcb,'X_o', '-118')
      |         set_param(gcb,'Y_o', '3.125')
      |         set_param(gcb,'Z_o', '0')
      |         set_param(gcb,'phi_o', '0')
      |         set_param(gcb,'theta_o', '0')
      |         set_param(gcb,'psi_o', '0')
      |     case 'Curved road'
      |         set_param(gcb,'X_o', '0.2')
      |         set_param(gcb,'Y_o', '-1605.0')
      |         set_param(gcb,'Z_o', '0')
      |         set_param(gcb,'phi_o', '0')
      |         set_param(gcb,'theta_o', '0')
      |         set_param(gcb,'psi_o', '-156*pi/180')
      |     case 'Parking lot'
      |         set_param(gcb,'X_o', '-104.0')
      |         set_param(gcb,'Y_o', '-9.7')
      |         set_param(gcb,'Z_o', '0')
      |         set_param(gcb,'phi_o', '0')
      |         set_param(gcb,'theta_o', '0')
      |         set_param(gcb,'psi_o', '0')
      |     case 'Double lane change'
      |         set_param(gcb,'X_o', '0')
      |         set_param(gcb,'Y_o', '3.125')
      |         set_param(gcb,'Z_o', '0')
      |         set_param(gcb,'phi_o', '0')
      |         set_param(gcb,'theta_o', '0')
      |         set_param(gcb,'psi_o', '0')
      |     case 'Open surface'
      |         set_param(gcb,'X_o', '0')
      |         set_param(gcb,'Y_o', '0')
      |         set_param(gcb,'Z_o', '0')
      |         set_param(gcb,'phi_o', '0')
      |         set_param(gcb,'theta_o', '0')
      |         set_param(gcb,'psi_o', '0')
      |     case 'US highway'
      |         set_param(gcb,'X_o', '3592.00')
      |         set_param(gcb,'Y_o', '2617.00')
      |         set_param(gcb,'Z_o', '-1.0')
      |         set_param(gcb,'phi_o', '0')
      |         set_param(gcb,'theta_o', '0')
      |         set_param(gcb,'psi_o', '0')
      |     case 'US city block'
      |         set_param(gcb,'X_o', '-125.19')
      |         set_param(gcb,'Y_o', '1.65')
      |         set_param(gcb,'Z_o', '-0.04')
      |         set_param(gcb,'phi_o', '0')
      |         set_param(gcb,'theta_o', '0')
      |         set_param(gcb,'psi_o', '0')
      |     case 'Large parking lot'
      |         set_param(gcb,'X_o', '45.0')
      |         set_param(gcb,'Y_o', '54.7')
      |         set_param(gcb,'Z_o', '0.0')
      |         set_param(gcb,'phi_o', '0')
      |         set_param(gcb,'theta_o', '0')
      |         set_param(gcb,'psi_o', '-pi/2')
      |     case 'Virtual Mcity'
      |         set_param(gcb,'X_o', '-26.0')
      |         set_param(gcb,'Y_o', '76.0')
      |         set_param(gcb,'Z_o', '0.0')
      |         set_param(gcb,'phi_o', '0')
      |         set_param(gcb,'theta_o', '0')
      |         set_param(gcb,'psi_o', '-40*pi/180')
      |     otherwise
      |         set_param(gcb,'X_o', '0')
      |         set_param(gcb,'Y_o', '0')
      |         set_param(gcb,'Z_o', '0')
      |         set_param(gcb,'phi_o', '0')
      |         set_param(gcb,'theta_o', '0')
      |         set_param(gcb,'psi_o', '0')
      | end
      | end
      mask TypeOptions defaultPos: Recommended for scene | User-specified
      mask DialogControl engineConfig Prompt: 3D Engine Settings
      mask DialogControl posSetup Prompt: Initial vehicle position
      mask DialogControl posSetupDesc Prompt: To use these initial vehicle positions, first Apply the initial values and then click Update the model workspaces with the initial values.
      mask DialogControl setModelPos Prompt: Update model workspaces with initial values
      mask DialogControl setModelPos Callback:
      | if strcmp(get_param(bdroot(gcb),'SimulationStatus'),'stopped')
      |     sceneType = get_param(gcb,'SceneDesc');
      |     rootModel = bdroot(gcb);
      |     ws = get_param(rootModel, 'modelworkspace');
      |     VEH = getVariable(ws,'VEH');
      |     ParamList={'X_o',[1,1],{};'Y_o',[1,1],{};'Z_o',[1,1],{};'phi_o',[1,1],{'gte',-pi/2;'lte',pi/2};'theta_o',[1,1],{'gte',-pi/2;'lte',pi/2};'psi_o',[1,1],{'gte',-2*pi;'lte',2*pi}};
      |     paramStruct = autoblkscheckparams(gcb, '3D Engine',ParamList);
      |     VEH.InitialLongPosition = paramStruct.X_o;
      |     VEH.InitialLatPosition = paramStruct.Y_o;
      |     VEH.InitialVertPosition = paramStruct.Z_o;
      |     VEH.InitialRollAngle = paramStruct.phi_o;
      |     VEH.InitialPitchAngle = paramStruct.theta_o;
      |     VEH.InitialYawAngle = paramStruct.psi_o;
      |     assignin(ws,'VEH',VEH);
      |     modelList = {'PassVeh14DOF','PassVeh7DOF'};
      |     for idx =1:length(modelList)
      | %         try
      |             load_system(modelList{idx});
      |             ws = get_param(modelList{idx}, 'modelworkspace');
      |             assignin(ws,'VEH',VEH);
      |             save_system(modelList{idx});
      |             close_system(modelList{idx});
      | %         catch
      | %             disp(['Cannot find ' modelList{idx}])
      | %         end
      |     end
      | end
      mask Display: disp('3D Engine')
  Acceleration Cmd : LinearGaugeBlock  LabelPosition=Hide  ScaleMax=1  TickInterval=0.20000000000000001
  Brake Cmd : LinearGaugeBlock  LabelPosition=Hide  ScaleMax=1  TickInterval=0.20000000000000001
  Bus Selector : BusSelector  Commented=on  OutputSignals=Driveline.EngSpd,Body.BdyFrm.Cg.Vel.xdot,Body.BdyFrm.Cg.Acc.ay
  Bus Selector1 : BusSelector  OutputSignals=Body.InertFrm.Cg.Ang.phi,Body.InertFrm.Cg.Ang.theta,Body.InertFrm.Cg.Ang.psi  OutputAsBus=on
  Bus Selector10 : BusSelector  OutputSignals=Wheels.signal1.TireFrame.Fx,Wheels.signal1.TireFrame.Fy
  Bus Selector2 : BusSelector  Commented=on  OutputSignals=Driver.AccFdbk,Driver.DecelFdbk,Driver.SteerFdbk
  Bus Selector3 : BusSelector  OutputSignals=Body.InertFrm.Cg.Disp.Y
  Bus Selector4 : BusSelector  Commented=on  OutputSignals=LeftBnd,RightBnd,LtrlRef
  Bus Selector5 : BusSelector  OutputSignals=Wheels.signal1.Steering.WhlAng  OutputAsBus=on
  Bus Selector6 : BusSelector  OutputSignals=Body.InertFrm.Geom.Disp.X,Body.InertFrm.Geom.Disp.Y,Body.InertFrm.Geom.Disp.Z  OutputAsBus=on
  Bus Selector7 : BusSelector  OutputSignals=Body.InertFrm.Geom.Vel.Xdot,Body.InertFrm.Geom.Vel.Ydot,Body.InertFrm.Geom.Vel.Zdot  OutputAsBus=on
  Bus Selector8 : BusSelector  OutputSignals=Body.InertFrm.Cg.Disp.X
  Bus Selector9 : BusSelector  Commented=on  OutputSignals=Driveline.EngSpd,Driveline.Gear  OutputAsBus=on
  Bus to Vector : BusToVector
  Bus to Vector1 : BusToVector
  Bus to Vector2 : BusToVector
  Bus to Vector3 : BusToVector  Commented=on
  Engine Tach [rpm] : CircularGaugeBlock  LabelPosition=Hide  ScaleMax=8000  TickInterval=1000
  Entered Gate : LampBlock  LabelPosition=Hide
  Ground1 : Ground
  Handwheel Angle [deg] : SemiCircularGaugeBlock  LabelPosition=Hide  ScaleMin=-300  ScaleMax=300  TickInterval=60
  ISO 15037-1:2006 : Subsystem  StopFcn=|  Variant=on  VariantControlMode=label  LabelModeActiveChoice=0  mask(ISO 15037-1:2006){Measurement=Disabled}
      | switch get_param(gcb,'Measurement')
      |     case 'Enabled'
      |        p=slproject.getCurrentProject;
      |        projectRoot=p.RootFolder;
      |        SySFolder=fullfile(projectRoot, 'System');
      |        Simulink.sdi.loadView([SySFolder filesep 'ISO15037_1_2006E.mldatx']);
      |        Simulink.sdi.view;
      | end
      mask prompts: Measurement "ISO Measurements"
      mask help: Enables display of ISO 15037-1:2006 standard measurement signals in the Simulation Data Inspector.
      mask init:
      | switch get_param(gcb,'Measurement')
      |     case 'Disabled'
      |         set_param(gcb,'OverrideUsingVariant','0')
      |     case 'Enabled'
      |        set_param(gcb,'OverrideUsingVariant','1')
      |     otherwise
      |        set_param(gcb,'OverrideUsingVariant','0')
      | end
      settings: AttributesFormatString=%<Measurement>
      mask Help: eval('vdynblkshelp(''iso15037'')');
      mask TypeOptions Measurement: Enabled | Disabled
      mask Callback Measurement:
      | switch get_param(gcb,'Measurement')
      |     case 'Disabled'
      |         set_param(gcb,'OverrideUsingVariant','0')
      |     case 'Enabled'
      |        set_param(gcb,'OverrideUsingVariant','1')
      |     otherwise
      |        set_param(gcb,'OverrideUsingVariant','0')
      | end
      mask Display: disp('ISO 15037-1:2006')
  Lane Change : Scope  Commented=on
  Lateral Acceleration [g] : SemiCircularGaugeBlock  LabelPosition=Hide  ScaleMin=-1  ScaleMax=1  TickInterval=0.5
  Mux : Mux  Inputs=3
  Mux1 : Mux  Commented=on
  Rate Transition : RateTransition  Commented=on  OutPortSampleTime=.1
  Rate Transition3 : RateTransition  Commented=on  OutPortSampleTime=.1
  Signal Specification : SignalSpecification  Commented=on  Unit=deg
  Signal Specification1 : SignalSpecification  Commented=on  Unit=mph
  Signal Specification2 : SignalSpecification  Commented=on  Unit=rpm
  Speed [mph] : CircularGaugeBlock  LabelPosition=Hide  TickInterval=10
  "Steer, Velocity, Lat Accel" : Scope  Commented=on  NumInputPorts=3
  Terminator{,1..3} (4 alike) : Terminator  Commented=on
  Unit Conversion1 : UnitConversion  Commented=on
  Unit Conversion2 : UnitConversion  Commented=on
  Unit Conversion3 : UnitConversion  Commented=on
  Vehicle XY Plotter : vehdynlibviscommon/Vehicle XY Plot Configuration  extRef=on  extStats=off  extTireF=on  a=VEH.FrontAxlePositionfromCG  b=VEH.RearAxlePositionfromCG  w=VEH.TrackWidth  figBorder=10  bufferSize=1024  velNorm=5  tireFNorm=1000  pltDT=.1
      settings: SourceProductBaseCode=VE
  wires:
  Signal Specification/1 -> "Steer, Velocity, Lat Accel"/1  "SteerAngle"
  Bus Selector/3 -> "Steer, Velocity, Lat Accel"/3  "<ay>"
  Bus Selector/2 -> "Steer, Velocity, Lat Accel"/2, Unit Conversion1/1  "<xdot>"
  Unit Conversion2/1 -> Signal Specification/1
  Unit Conversion1/1 -> Signal Specification1/1
  Signal Specification1/1 -> Terminator/1  "xdot_mph"
  Bus Selector4/2 -> Rate Transition3/1  "<RightBnd>"
  Mux1/1 -> Lane Change/1
  Bus Selector3/1 -> Mux1/4  "<Y>"
  Bus Selector4/1 -> Rate Transition/1  "<LeftBnd>"
  Bus Selector4/3 -> Mux1/3  "<LtrlRef>"
  Bus Selector2/3 -> Unit Conversion2/1  "<SteerFdbk>"
  Bus Selector2/1 -> Terminator1/1  "<AccFdbk>"
  Bus Selector2/2 -> Terminator2/1  "<DecelFdbk>"
  Signal Specification2/1 -> Terminator3/1  "Engine_rpm"
  Unit Conversion3/1 -> Signal Specification2/1
  Bus Selector/1 -> Unit Conversion3/1  "<EngSpd>"
  Bus Selector7/1 -> Bus to Vector1/1
  Bus to Vector/1 -> Vehicle XY Plotter/1
  Bus Selector6/1 -> Bus to Vector/1
  Bus to Vector1/1 -> Vehicle XY Plotter/3
  Bus Selector1/1 -> Bus to Vector2/1
  Bus Element In2/1 -> ISO 15037-1:2006/1(VehFdbk), Bus Selector10/1, Bus Selector9/1, Bus Selector8/1, Bus Selector5/1, Bus Selector7/1, Bus Selector1/1, Bus Selector6/1, 3D Engine/1(VehFdbk), Bus Selector3/1, Bus Selector2/1, Bus Selector/1  "VehFdbk"
  Mux/1 -> Vehicle XY Plotter/5
  Ground1/1 -> Mux/3
  Bus Element In/1 -> Bus Selector4/1
  Bus Element In1/1 -> ?
  Bus to Vector3/1 -> ?
  Bus Selector9/1 -> Bus to Vector3/1
  Bus to Vector2/1 -> Vehicle XY Plotter/2
  Bus Selector5/1 -> Vehicle XY Plotter/4
  Bus Selector10/2 -> Vehicle XY Plotter/7  "<Fy>"
  Bus Selector10/1 -> Vehicle XY Plotter/6  "<Fx>"
  Rate Transition/1 -> Mux1/1  "Left Boundary"
  Rate Transition3/1 -> Mux1/2  "Right Boundary"
  [yRef] -> Mux/2
  [xRef] -> Mux/1

== system vehicle_model/lateral controller ==
  vehfdbk1 : Inport
  long_ref : Inport  Port=2
  Bus Selector : BusSelector  OutputSignals=Body.BdyFrm.Cg.Vel.xdot,Body.BdyFrm.Cg.AngVel.r
  Degrees to Radians1 : simulink_extras/Transformations/Degrees to Radians
  Gain : Gain  Gain=18
  Lateral Controller Stanley : drivingvehiclecontroller/Lateral Controller Stanley  ModelType=Dynamic bicycle model  PositionGainF=2.5  PositionGainR=2.5  YawRateGain=0.2  DelayGain=0.2  VehicleMass=VEH.Mass  Lf=VEH.FrontAxlePositionfromCG  Lr=VEH.RearAxlePositionfromCG  TireStiffness=2*0.7*4.5e4  Wheelbase=3  MaxSteeringAngle=45
      settings: SourceProductBaseCode=DR
  Radians to Degrees : simulink_extras/Transformations/Radians to Degrees
  Rate Transition : RateTransition
  Reference Data : Subsystem  VariantControl=Stanley
  Saturation : Saturate  UpperLimit=inf  LowerLimit=0.1
  Subsystem : Subsystem
  Unit Delay : UnitDelay  SampleTime=-1  HasFrameUpgradeWarning=on
  Steer_cmd : Outport
  wires:
  Bus Selector/1 -> Saturation/1  "<xdot>"
  vehfdbk1/1 -> Bus Selector/1, Subsystem/1(VehFdbk)
  Reference Data/2(DirectionO) -> Lateral Controller Stanley/4
  Rate Transition/1 -> Steer_cmd/1
  Gain/1 -> Rate Transition/1
  Lateral Controller Stanley/1 -> Unit Delay/1, Degrees to Radians1/1
  Bus Selector/2 -> Radians to Degrees/1  "<r>"
  Subsystem/1(pose) -> Lateral Controller Stanley/2
  Reference Data/1(RefPose) -> Lateral Controller Stanley/1
  Degrees to Radians1/1 -> Gain/1
  Saturation/1 -> Reference Data/2(VelFdbk), Lateral Controller Stanley/3
  long_ref/1 -> Reference Data/1(long_ref)
  Radians to Degrees/1 -> ?
  Reference Data/3(CurvatureO) -> ?
  Unit Delay/1 -> ?

== system vehicle_model/Controllers/Powertrain Control Input ==
  OpCmds : Inport
  VehPlnt : Inport  Port=2
  Bus Selector1 : BusSelector  OutputSignals=Veh.xdot,Veh.MotSpd,Elec.BMS_Sensors
  Bus Selector2 : BusSelector  OutputSignals=AccelCmd,DecelCmd
  Rate Transition : RateTransition  Deterministic=off
  Rate Transition1 : RateTransition  Deterministic=off
  Rate Transition2 : RateTransition  Deterministic=off  OutPortSampleTimeOpt=Inherit
  Rate Transition6 : RateTransition  Deterministic=off  OutPortSampleTimeOpt=Inherit
  AccelPdl : Outport  VectorParamsAs1DForOutWhenUnconnected=off
  DecelPdl : Outport  Port=2  VectorParamsAs1DForOutWhenUnconnected=off
  VehSpdFdbk : Outport  Port=3  VectorParamsAs1DForOutWhenUnconnected=off
  MotSpd : Outport  Port=4  VectorParamsAs1DForOutWhenUnconnected=off
  BMS_Sensors : Outport  Port=5  OutDataTypeStr=Bus: Sensors  VectorParamsAs1DForOutWhenUnconnected=off
  wires:
  OpCmds/1 -> Bus Selector2/1
  VehPlnt/1 -> Bus Selector1/1
  Bus Selector2/1 -> Rate Transition/1  "<AccelCmd>"
  Bus Selector2/2 -> Rate Transition1/1  "<DecelCmd>"
  Bus Selector1/1 -> Rate Transition2/1  "<xdot>"
  Bus Selector1/2 -> Rate Transition6/1  "<MotSpd>"
  Rate Transition/1 -> AccelPdl/1
  Rate Transition1/1 -> DecelPdl/1
  Rate Transition2/1 -> VehSpdFdbk/1
  Rate Transition6/1 -> MotSpd/1
  Bus Selector1/3 -> BMS_Sensors/1  "<BMS_Sensors>"

== system vehicle_model/Controllers/Powertrain Control Module (PCM) ==
  AccCmd : Inport
  DecCmd : Inport  Port=2
  VehSpdFdbk : Inport  Port=3
  MotSpd : Inport  Port=4
  BMS_Sensors : Inport  Port=5  OutDataTypeStr=Bus: Sensors
  Subsystem : Subsystem
  Subsystem1 : Subsystem
  MotTrqCmd : Outport
  BrakeCmd : Outport  Port=2
  BMS_Info : Outport  Port=3  OutDataTypeStr=Bus: SOC_Est
  BMS_Cmd : Outport  Port=4  OutDataTypeStr=Bus: CurrentLimits
  wires:
  DecCmd/1 -> Subsystem1/2(DecCmd)
  Subsystem1/1(MotTrqCmd) -> MotTrqCmd/1
  [BMS_Info] -> Subsystem1/4(Batt_Info)
  MotSpd/1 -> Subsystem1/6(MotSpd)
  VehSpdFdbk/1 -> Subsystem1/3(VehSpdFdbk)
  AccCmd/1 -> Subsystem1/1(AccCmd)
  Subsystem1/2(BrakeCmd) -> BrakeCmd/1
  Subsystem/1(BMS_Info) -> [BMS_Info], BMS_Info/1
  Subsystem/2(BMS_Cmd) -> BMS_Cmd/1, [BMS_Cmd]
  BMS_Sensors/1 -> Subsystem/1(Sensors), Subsystem1/7(BMS_Sensors)
  [BMS_Cmd] -> Subsystem1/5(BMS_Cmd)

== system vehicle_model/Controllers/Powertrain Control Output ==
  MotTrqCmd : Inport
  BrkCmd : Inport  Port=2
  BMS_Info : Inport  Port=3  OutDataTypeStr=Bus: SOC_Est
  BMS_Cmd : Inport  Port=4  OutDataTypeStr=Bus: CurrentLimits
  Bus Creator : BusCreator  Inputs=4
  PtCtrl : Outport  VectorParamsAs1DForOutWhenUnconnected=off
  wires:
  BrkCmd/1 -> Bus Creator/2  "BrkCmd"
  Bus Creator/1 -> PtCtrl/1  "PtCtrl"
  MotTrqCmd/1 -> Bus Creator/1  "MotTrqCmd"
  BMS_Info/1 -> Bus Creator/3  "BMS_Info"
  BMS_Cmd/1 -> Bus Creator/4  "BMS_Cmd"

== system vehicle_model/Passenger Car/Drivetrain Output ==
  Vel : Inport
  MotSpd : Inport  Port=2
  Bus Creator1 : BusCreator  Inputs=2
  VehFdbk : Outport  VectorParamsAs1DForOutWhenUnconnected=off
  wires:
  Bus Creator1/1 -> VehFdbk/1  "VehFdbk"
  MotSpd/1 -> Bus Creator1/2  "MotSpd"
  Vel/1 -> Bus Creator1/1

== system vehicle_model/Passenger Car/Drivetrain Plant Input ==
  Ctrl : Inport
  ElecFdbk : Inport  Port=2
  Env : Inport  Port=3
  Driver : Inport  Port=4
  Bus Selector : BusSelector  OutputSignals=BrkCmd
  Bus Selector1 : BusSelector  OutputSignals=MotTrq
  Bus Selector2 : BusSelector  OutputSignals=Ground.Ground_mu,Wind,Ground.z
  Bus Selector3 : BusSelector  Commented=on  OutputSignals=Ground.Grade,Wind.wind_x
  Bus Selector4 : BusSelector  OutputSignals=SteerCmd
  First Order Hold : FirstOrderHold  ErrorTolerance=inf
  Rate Transition6 : RateTransition  Commented=on  Deterministic=off
  Rate Transition7 : RateTransition  Commented=on  Deterministic=off
  MotTrq : Outport  VectorParamsAs1DForOutWhenUnconnected=off
  BrkCmd : Outport  Port=2  VectorParamsAs1DForOutWhenUnconnected=off
  Grade : Outport  Port=3  VectorParamsAs1DForOutWhenUnconnected=off
  WindVel : Outport  Port=4  VectorParamsAs1DForOutWhenUnconnected=off
  mu : Outport  Port=5
  Gnd : Outport  Port=6
  Steer : Outport  Port=7
  wires:
  Ctrl/1 -> Bus Selector/1
  Bus Selector/1 -> First Order Hold/1  "<BrkCmd>"
  ElecFdbk/1 -> Bus Selector1/1
  Bus Selector1/1 -> MotTrq/1  "<MotTrq>"
  Env/1 -> Bus Selector2/1, Bus Selector3/1
  Rate Transition6/1 -> Grade/1  "Grade"
  Rate Transition7/1 -> ?  "WindVel"
  Bus Selector3/1 -> Rate Transition6/1  "<Grade>"
  Bus Selector3/2 -> Rate Transition7/1  "<wind_x>"
  Bus Selector2/2 -> WindVel/1  "<Wind>"
  Bus Selector2/1 -> mu/1  "<Ground_mu>"
  Bus Selector2/3 -> Gnd/1  "<z>"
  Driver/1 -> Bus Selector4/1
  Bus Selector4/1 -> Steer/1  "<SteerCmd>"
  First Order Hold/1 -> BrkCmd/1

== system vehicle_model/Passenger Car/Electric Plant Input ==
  Ctrl : Inport
  Veh : Inport  Port=2
  Env : Inport  Port=3
  Bus Selector : BusSelector  OutputSignals=MotTrqCmd,BMS_Info,BMS_Cmd
  Bus Selector1 : BusSelector  OutputSignals=MotSpd
  Bus Selector2 : BusSelector  OutputSignals=Temp
  First Order Hold : FirstOrderHold  ErrorTolerance=inf  AllowContinuousInput=on
  Zero-Order Hold1 : ZeroOrderHold  Commented=on  SampleTime=-1
  MotTrqCmd : Outport  VectorParamsAs1DForOutWhenUnconnected=off
  MotSpd : Outport  Port=2  VectorParamsAs1DForOutWhenUnconnected=off
  AmbTmp : Outport  Port=3  VectorParamsAs1DForOutWhenUnconnected=off
  BMS_Info : Outport  Port=4  VectorParamsAs1DForOutWhenUnconnected=off
  wires:
  First Order Hold/1 -> MotTrqCmd/1  "MotTrqCmd"
  Ctrl/1 -> Bus Selector/1
  Bus Selector/1 -> First Order Hold/1  "<MotTrqCmd>"
  Veh/1 -> Bus Selector1/1
  Bus Selector1/1 -> MotSpd/1  "<MotSpd>"
  Env/1 -> Bus Selector2/1
  Bus Selector2/1 -> AmbTmp/1  "<Temp>"
  Bus Selector/2 -> BMS_Info/1  "<BMS_Info>"

== system vehicle_model/Passenger Car/Electric Plant Output ==
  BattSoc : Inport
  BattPwr : Inport  Port=2
  BattCrnt : Inport  Port=3
  MotTrq : Inport  Port=4
  BMS_Sensors : Inport  Port=5  OutDataTypeStr=Bus: Sensors
  Bus Creator1 : BusCreator  Inputs=5
  ElecFdbk : Outport  VectorParamsAs1DForOutWhenUnconnected=off
  wires:
  Bus Creator1/1 -> ElecFdbk/1  "ElecFdbk"
  BattPwr/1 -> Bus Creator1/2
  BattCrnt/1 -> Bus Creator1/3
  MotTrq/1 -> Bus Creator1/4
  BattSoc/1 -> Bus Creator1/1
  BMS_Sensors/1 -> Bus Creator1/5

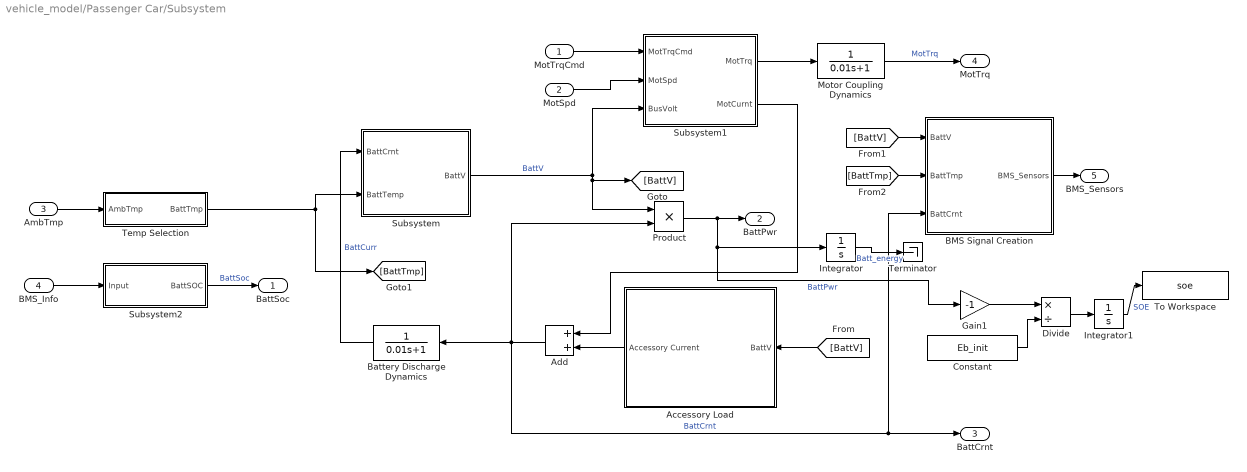
== system vehicle_model/Passenger Car/Subsystem ==
  MotTrqCmd : Inport
  MotSpd : Inport  Port=2
  AmbTmp : Inport  Port=3
  BMS_Info : Inport  Port=4
  Accessory Load : Subsystem
  Add : Sum
  BMS Signal Creation : Subsystem
  Battery Discharge Dynamics : TransferFcn  Denominator=[0.01 1]
  Constant : Constant  Value=Eb_init
  Divide : Product  Inputs=*/
  Gain1 : Gain  Gain=-1
  Integrator : Integrator  InitialCondition=Eb_init*SOE_init
  Integrator1 : Integrator  InitialCondition=SOE_init
  Motor Coupling Dynamics : TransferFcn  Denominator=[0.01 1]
  Product : Product
  Subsystem : Subsystem
  Subsystem1 : Subsystem
  Subsystem2 : Subsystem
  Temp Selection : Subsystem
  Terminator : Terminator
  To Workspace : ToWorkspace  VariableName=soe  SaveFormat=Timeseries  SampleTime=-1
  BattSoc : Outport
  BattPwr : Outport  Port=2  VectorParamsAs1DForOutWhenUnconnected=off
  BattCrnt : Outport  Port=3  VectorParamsAs1DForOutWhenUnconnected=off
  MotTrq : Outport  Port=4  VectorParamsAs1DForOutWhenUnconnected=off
  BMS_Sensors : Outport  Port=5  OutDataTypeStr=Bus: Sensors  VectorParamsAs1DForOutWhenUnconnected=off
  wires:
  Subsystem1/2(MotCurnt) -> Add/1
  MotTrqCmd/1 -> Subsystem1/1(MotTrqCmd)
  MotSpd/1 -> Subsystem1/2(MotSpd)
  Battery Discharge Dynamics/1 -> Subsystem/1(BattCrnt)  "BattCurr"
  Subsystem/1(BattV) -> Subsystem1/3(BusVolt), Product/1, [BattV]  "BattV"
  [BattTmp] -> BMS Signal Creation/2(BattTmp)
  BMS_Info/1 -> Subsystem2/1(Input)
  Subsystem2/1(BattSOC) -> BattSoc/1  "BattSoc"
  Add/1 -> Battery Discharge Dynamics/1, BattCrnt/1, BMS Signal Creation/3(BattCrnt), Product/2  "BattCrnt"
  [BattV] -> Accessory Load/1(BattV)
  BMS Signal Creation/1(BMS_Sensors) -> BMS_Sensors/1
  [BattV] -> BMS Signal Creation/1(BattV)
  Subsystem1/1(MotTrq) -> Motor Coupling Dynamics/1
  AmbTmp/1 -> Temp Selection/1(AmbTmp)
  Temp Selection/1(BattTmp) -> Subsystem/2(BattTemp), [BattTmp]
  Accessory Load/1(Accessory Current) -> Add/2
  Motor Coupling Dynamics/1 -> MotTrq/1  "MotTrq"
  Integrator/1 -> Terminator/1  "Batt_energy"
  Constant/1 -> Divide/2
  Integrator1/1 -> To Workspace/1  "SOE"
  Product/1 -> Gain1/1, Integrator/1, BattPwr/1  "BattPwr"
  Divide/1 -> Integrator1/1
  Gain1/1 -> Divide/1
